simulink model "teste_FT"  (R2023a)
settings: Solver=VariableStepAuto  StartTime=0.0  StopTime=125  RelTol=1e-3
settings Model: Creator=Maria  LastModifiedBy=Maria

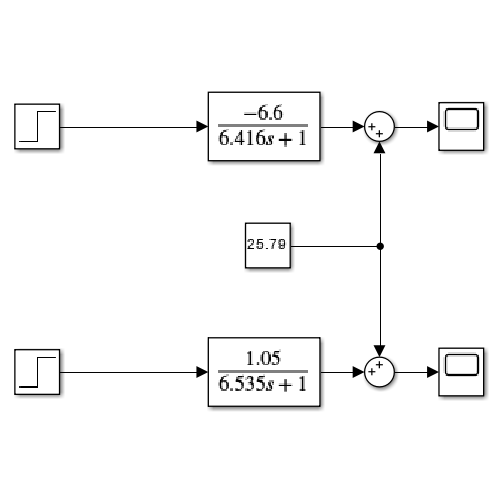
[thumbnail: Simulink's stored preview of the top-level diagram]
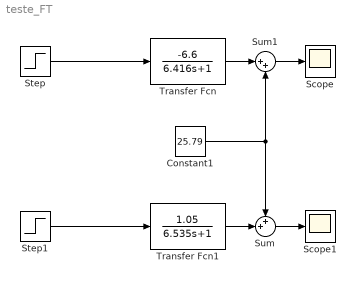
== system teste_FT ==
  Constant1 : Constant  Value=25.79
  Scope : Scope
  Scope1 : Scope
  Step : Step  Time=75  After=0.05  SampleTime=0
  Step1 : Step  Time=50  SampleTime=0
  Sum : Sum  Inputs=++|
  Sum1 : Sum  Inputs=|++
  Transfer Fcn : TransferFcn  Numerator=[-6.6]  Denominator=[6.416 1]
  Transfer Fcn1 : TransferFcn  Numerator=[1.05]  Denominator=[6.535 1]
  wires:
  Step/1 -> Transfer Fcn/1
  Step1/1 -> Transfer Fcn1/1
  Sum/1 -> Scope1/1
  Transfer Fcn/1 -> Sum1/1
  Sum1/1 -> Scope/1
  Constant1/1 -> Sum1/2, Sum/1
  Transfer Fcn1/1 -> Sum/2
